simulink model "Turbulence_VonKarman"  (R2014a)
settings: Solver=ode4  StartTime=0.0  StopTime=time  FixedStep=0.02  RelTol=1e-3
PreLoadFcn:
  | load init.mat;
values from neighbouring files (symbols this model uses):
  altitude_worst = 150    [Main_turbulence_vonKarman.m]    (also in compute_variance.m)
  Vc_max = 5    [Main_turbulence_vonKarman.m]    (also in compute_variance.m)
  Vc_min = -5    [Main_turbulence_vonKarman.m]    (also in compute_variance.m)
  Vcruise = 30    [Main_turbulence_vonKarman.m]    (also in compute_variance.m)
undefined symbols (not defined in the file or in its folder): turbulenceParameters
libraries: simulink x3, aerolibconvert2 x3
settings Model: Creator=Piero  LastModifiedBy=Domenico

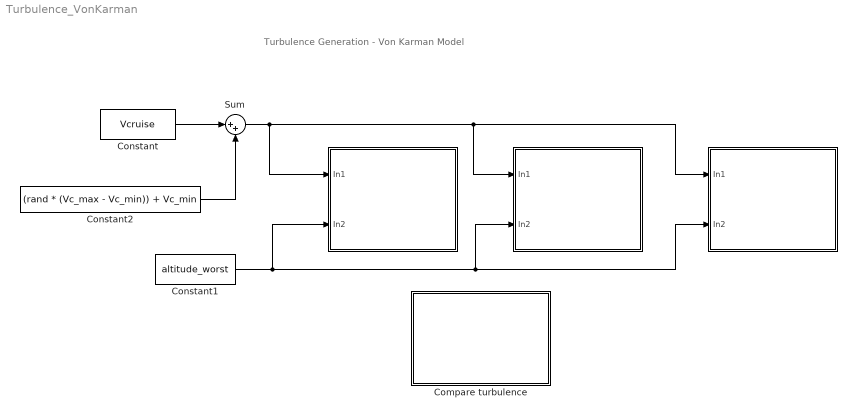
== system Turbulence_VonKarman ==
  note: Turbulence Generation - Von Karman Model
  " " : Subsystem
      mask Display:
      | color('green');
      | disp('Light Turbulence')
      | color('black');
      | port_label('input',1,'Airspeed [m/s]','texmode', 'on')
      | port_label('input',2,'Altitude [m]')
  "   " : Subsystem
      mask Display:
      | color('green');
      | disp('Moderate Turbulence')
      | color('black');
      | port_label('input',1,'Airspeed [m/s]','texmode', 'on')
      | port_label('input',2,'Altitude [m]')
  "      " : Subsystem
      mask Display:
      | color('green');
      | disp('Heavy Turbulence')
      | color('black');
      | port_label('input',1,'Airspeed [m/s]','texmode', 'on')
      | port_label('input',2,'Altitude [m]')
  " Compare turbulence" : Subsystem
      mask Display:
      | color('red');
      | disp('Plot section')
  Constant : Constant  Value=Vcruise
  Constant1 : Constant  Value=altitude_worst
  Constant2 : Constant  Value=(rand * (Vc_max - Vc_min)) + Vc_min
  Sum : Sum  Inputs=|++
  wires:
  Constant1/1 -> "      "/2(In2), "   "/2(In2), " "/2(In2)
  Sum/1 -> " "/1(In1), "   "/1(In1), "      "/1(In1)
  Constant/1 -> Sum/1
  Constant2/1 -> Sum/2

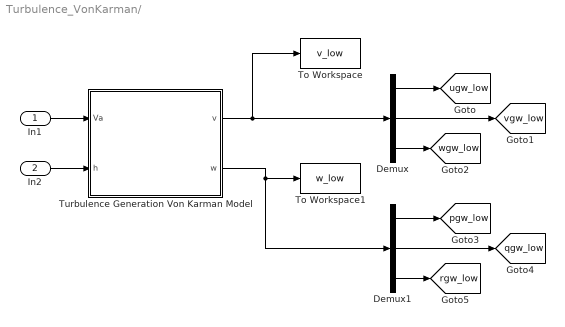
== system Turbulence_VonKarman/  ==
  In1 : Inport
  In2 : Inport  Port=2
  Demux : Demux  Outputs=3
  Demux1 : Demux  Outputs=3
  To Workspace : ToWorkspace  VariableName=v_low  SaveFormat=Structure With Time  SampleTime=-1
  To Workspace1 : ToWorkspace  VariableName=w_low  SaveFormat=Structure With Time  SampleTime=-1
  "Turbulence Generation Von Karman Model " : Subsystem  mask{ts=Light}
      mask prompts: ts "Turbulence Severity"
      mask TypeOptions ts: Light | Moderate | Heavy
      mask DialogControl DescTextVar Prompt: Generates the wind turbulences according to Dryden equations
      mask Display:
      | color('red');
      | disp('Turbulence\n Generation')
      | color('black');
      | port_label('output',1,'v_{wind}','texmode', 'on')
      | port_label('output',2,'\omega_{wind}','texmode', 'on')
      | 
      | port_label('input',1,'Airspeed')
      | port_label('input',2,'Altitude')
  tag scope: pgw_low=global, qgw_low=global, rgw_low=global, ugw_low=global, vgw_low=global, wgw_low=global
  wires:
  Demux/1 -> [ugw_low]
  Demux/2 -> [vgw_low]
  In1/1 -> "Turbulence Generation Von Karman Model "/1(Va)
  "Turbulence Generation Von Karman Model "/1(v) -> To Workspace/1, Demux/1
  "Turbulence Generation Von Karman Model "/2(w) -> To Workspace1/1, Demux1/1
  Demux1/1 -> [pgw_low]
  Demux1/2 -> [qgw_low]
  Demux1/3 -> [rgw_low]
  Demux/3 -> [wgw_low]
  In2/1 -> "Turbulence Generation Von Karman Model "/2(h)

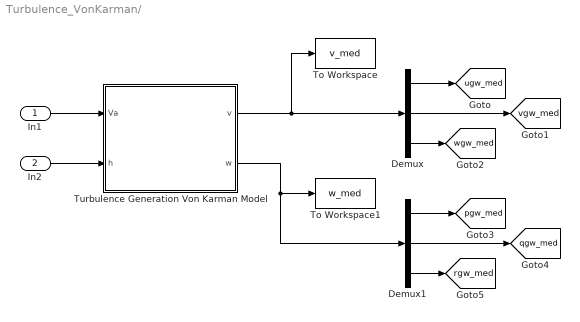
== system Turbulence_VonKarman/    ==
  In1 : Inport
  In2 : Inport  Port=2
  Demux : Demux  Outputs=3
  Demux1 : Demux  Outputs=3
  To Workspace : ToWorkspace  VariableName=v_med  SaveFormat=Structure With Time  SampleTime=-1
  To Workspace1 : ToWorkspace  VariableName=w_med  SaveFormat=Structure With Time  SampleTime=-1
  "Turbulence Generation Von Karman Model " : Subsystem  mask{ts=Moderate}
      mask prompts: ts "Turbulence Severity"
      mask TypeOptions ts: Light | Moderate | Heavy
      mask DialogControl DescTextVar Prompt: Generates the wind turbulences according to Dryden equations
      mask Display:
      | color('red');
      | disp('Turbulence\n Generation')
      | color('black');
      | port_label('output',1,'v_{wind}','texmode', 'on')
      | port_label('output',2,'\omega_{wind}','texmode', 'on')
      | 
      | port_label('input',1,'Airspeed')
      | port_label('input',2,'Altitude')
  tag scope: pgw_med=global, qgw_med=global, rgw_med=global, ugw_med=global, vgw_med=global, wgw_med=global
  wires:
  Demux/3 -> [wgw_med]
  Demux1/3 -> [rgw_med]
  Demux1/2 -> [qgw_med]
  Demux1/1 -> [pgw_med]
  "Turbulence Generation Von Karman Model "/2(w) -> To Workspace1/1, Demux1/1
  "Turbulence Generation Von Karman Model "/1(v) -> To Workspace/1, Demux/1
  Demux/2 -> [vgw_med]
  Demux/1 -> [ugw_med]
  In1/1 -> "Turbulence Generation Von Karman Model "/1(Va)
  In2/1 -> "Turbulence Generation Von Karman Model "/2(h)

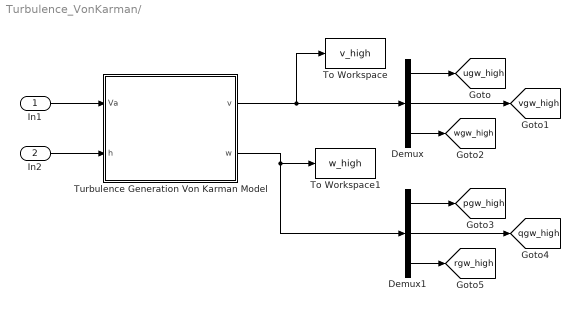
== system Turbulence_VonKarman/       ==
  In1 : Inport
  In2 : Inport  Port=2
  Demux : Demux  Outputs=3
  Demux1 : Demux  Outputs=3
  To Workspace : ToWorkspace  VariableName=v_high  SaveFormat=Structure With Time  SampleTime=-1
  To Workspace1 : ToWorkspace  VariableName=w_high  SaveFormat=Structure With Time  SampleTime=-1
  "Turbulence Generation Von Karman Model " : Subsystem  mask{ts=Heavy}
      mask prompts: ts "Turbulence Severity"
      mask TypeOptions ts: Light | Moderate | Heavy
      mask DialogControl DescTextVar Prompt: Generates the wind turbulences according to Dryden equations
      mask Display:
      | color('red');
      | disp('Turbulence\n Generation')
      | color('black');
      | port_label('output',1,'v_{wind}','texmode', 'on')
      | port_label('output',2,'\omega_{wind}','texmode', 'on')
      | 
      | port_label('input',1,'Airspeed')
      | port_label('input',2,'Altitude')
  tag scope: pgw_high=global, qgw_high=global, rgw_high=global, ugw_high=global, vgw_high=global, wgw_high=global
  wires:
  Demux/1 -> [ugw_high]
  Demux/2 -> [vgw_high]
  In2/1 -> "Turbulence Generation Von Karman Model "/2(h)
  "Turbulence Generation Von Karman Model "/1(v) -> To Workspace/1, Demux/1
  "Turbulence Generation Von Karman Model "/2(w) -> To Workspace1/1, Demux1/1
  Demux1/1 -> [pgw_high]
  Demux1/2 -> [qgw_high]
  Demux1/3 -> [rgw_high]
  Demux/3 -> [wgw_high]
  In1/1 -> "Turbulence Generation Von Karman Model "/1(Va)

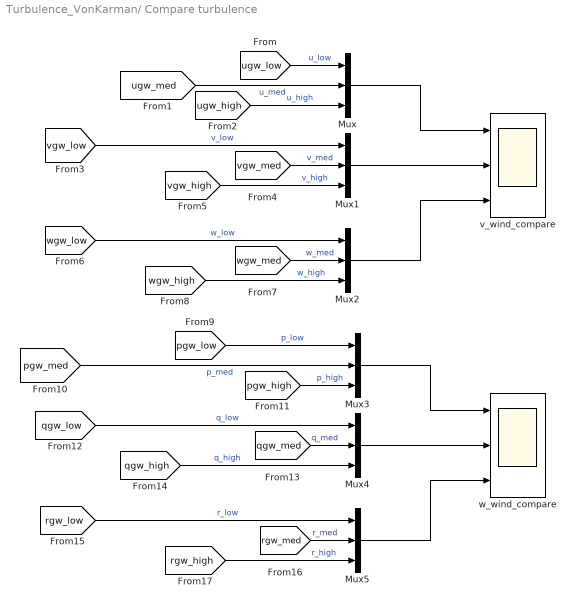
== system Turbulence_VonKarman/ Compare turbulence ==
  Mux{,1..5} (6 alike) : Mux  Inputs=3
  v_wind_compare : Scope  NumInputPorts=3
      settings: ShowLegends=on  YMin=-5~-5~-5  YMax=5~5~5  SaveName=V_wind_compare  SampleTime=0.01
  w_wind_compare : Scope  NumInputPorts=3
      settings: ShowLegends=on  YMin=-5~-5~-5  YMax=5~5~5  SaveName=w_wind_compare  SampleTime=0.01
  wires:
  [wgw_low] -> Mux2/1  "w_low"
  [ugw_med] -> Mux/2  "u_med"
  Mux/1 -> v_wind_compare/1
  [wgw_high] -> Mux2/3  "w_high"
  Mux2/1 -> v_wind_compare/3
  [vgw_med] -> Mux1/2  "v_med"
  [ugw_low] -> Mux/1  "u_low"
  [vgw_low] -> Mux1/1  "v_low"
  [vgw_high] -> Mux1/3  "v_high"
  Mux1/1 -> v_wind_compare/2
  [wgw_med] -> Mux2/2  "w_med"
  [ugw_high] -> Mux/3  "u_high"
  [qgw_med] -> Mux4/2  "q_med"
  [qgw_high] -> Mux4/3  "q_high"
  [rgw_low] -> Mux5/1  "r_low"
  [rgw_med] -> Mux5/2  "r_med"
  [rgw_high] -> Mux5/3  "r_high"
  [pgw_low] -> Mux3/1  "p_low"
  Mux3/1 -> w_wind_compare/1
  Mux4/1 -> w_wind_compare/2
  Mux5/1 -> w_wind_compare/3
  [pgw_med] -> Mux3/2  "p_med"
  [pgw_high] -> Mux3/3  "p_high"
  [qgw_low] -> Mux4/1  "q_low"

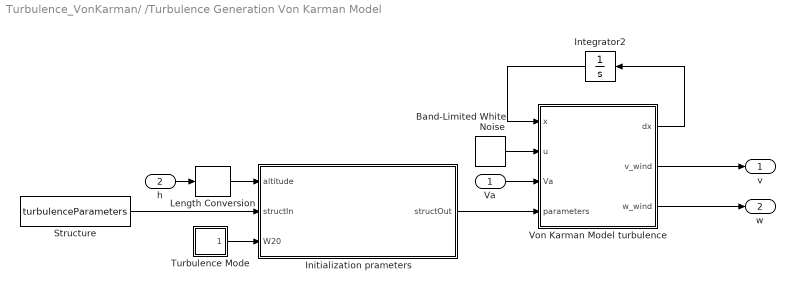
== system Turbulence_VonKarman/ /Turbulence Generation Von Karman Model  ==
  Va : Inport
  h : Inport  Port=2
  Band-Limited White Noise : simulink/Sources/Band-Limited White Noise  Cov=[0.1]  Ts=0.02  seed=[23341]
  Initialization prameters : MATLAB Function  TreatAsAtomicUnit=on
  Integrator2 : Integrator  InitialCondition=zeros(17,1)
  Length Conversion : aerolibconvert2/Length Conversion  IU=m  OU=ft
  Structure : Constant  Value=turbulenceParameters  OutDataTypeStr=Bus: myTurbParams
  Turbulence Mode : Subsystem
  Von Karman Model turbulence : MATLAB Function  TreatAsAtomicUnit=on
  v : Outport
  w : Outport  Port=2
  wires:
  h/1 -> Length Conversion/1
  Structure/1 -> Initialization prameters/2(structIn)
  Length Conversion/1 -> Initialization prameters/1(altitude)
  Va/1 -> Von Karman Model turbulence/3(Va)
  Integrator2/1 -> Von Karman Model turbulence/1(x)
  Von Karman Model turbulence/1(dx) -> Integrator2/1
  Band-Limited White Noise/1 -> Von Karman Model turbulence/2(u)
  Von Karman Model turbulence/3(w_wind) -> w/1
  Von Karman Model turbulence/2(v_wind) -> v/1
  Initialization prameters/1(structOut) -> Von Karman Model turbulence/4(parameters)
  Turbulence Mode/1(W20) -> Initialization prameters/3(W20)

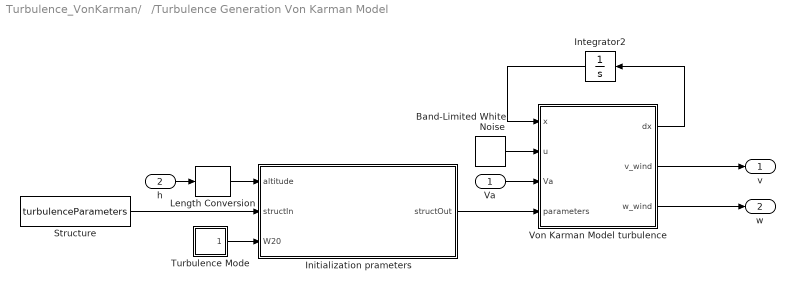
== system Turbulence_VonKarman/   /Turbulence Generation Von Karman Model  ==
  Va : Inport
  h : Inport  Port=2
  Band-Limited White Noise : simulink/Sources/Band-Limited White Noise  Cov=[0.1]  Ts=0.02  seed=[23341]
  Initialization prameters : MATLAB Function  TreatAsAtomicUnit=on
  Integrator2 : Integrator  InitialCondition=zeros(17,1)
  Length Conversion : aerolibconvert2/Length Conversion  IU=m  OU=ft
  Structure : Constant  Value=turbulenceParameters  OutDataTypeStr=Bus: myTurbParams
  Turbulence Mode : Subsystem
  Von Karman Model turbulence : MATLAB Function  TreatAsAtomicUnit=on
  v : Outport
  w : Outport  Port=2
  wires:
  Turbulence Mode/1(W20) -> Initialization prameters/3(W20)
  Initialization prameters/1(structOut) -> Von Karman Model turbulence/4(parameters)
  Von Karman Model turbulence/2(v_wind) -> v/1
  Von Karman Model turbulence/3(w_wind) -> w/1
  Band-Limited White Noise/1 -> Von Karman Model turbulence/2(u)
  Von Karman Model turbulence/1(dx) -> Integrator2/1
  Integrator2/1 -> Von Karman Model turbulence/1(x)
  Va/1 -> Von Karman Model turbulence/3(Va)
  Length Conversion/1 -> Initialization prameters/1(altitude)
  Structure/1 -> Initialization prameters/2(structIn)
  h/1 -> Length Conversion/1

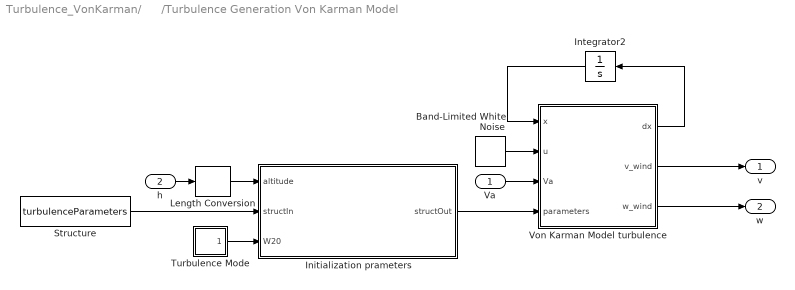
== system Turbulence_VonKarman/      /Turbulence Generation Von Karman Model  ==
  Va : Inport
  h : Inport  Port=2
  Band-Limited White Noise : simulink/Sources/Band-Limited White Noise  Cov=[0.1]  Ts=0.02  seed=[23341]
  Initialization prameters : MATLAB Function  TreatAsAtomicUnit=on
  Integrator2 : Integrator  InitialCondition=zeros(17,1)
  Length Conversion : aerolibconvert2/Length Conversion  IU=m  OU=ft
  Structure : Constant  Value=turbulenceParameters  OutDataTypeStr=Bus: myTurbParams
  Turbulence Mode : Subsystem
  Von Karman Model turbulence : MATLAB Function  TreatAsAtomicUnit=on
  v : Outport
  w : Outport  Port=2
  wires:
  h/1 -> Length Conversion/1
  Structure/1 -> Initialization prameters/2(structIn)
  Length Conversion/1 -> Initialization prameters/1(altitude)
  Va/1 -> Von Karman Model turbulence/3(Va)
  Integrator2/1 -> Von Karman Model turbulence/1(x)
  Von Karman Model turbulence/1(dx) -> Integrator2/1
  Band-Limited White Noise/1 -> Von Karman Model turbulence/2(u)
  Von Karman Model turbulence/3(w_wind) -> w/1
  Von Karman Model turbulence/2(v_wind) -> v/1
  Initialization prameters/1(structOut) -> Von Karman Model turbulence/4(parameters)
  Turbulence Mode/1(W20) -> Initialization prameters/3(W20)

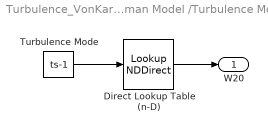
== system Turbulence_VonKarman/ /Turbulence Generation Von Karman Model /Turbulence Mode ==
  Direct Lookup Table (n-D) : LookupNDDirect  NumberOfTableDimensions=1  Table=[15 30 45]
  Turbulence Mode : Constant  Value=ts-1
  W20 : Outport
  wires:
  Direct Lookup Table (n-D)/1 -> W20/1
  Turbulence Mode/1 -> Direct Lookup Table (n-D)/1

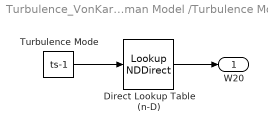
== system Turbulence_VonKarman/   /Turbulence Generation Von Karman Model /Turbulence Mode ==
  Direct Lookup Table (n-D) : LookupNDDirect  NumberOfTableDimensions=1  Table=[15 30 45]
  Turbulence Mode : Constant  Value=ts-1
  W20 : Outport
  wires:
  Turbulence Mode/1 -> Direct Lookup Table (n-D)/1
  Direct Lookup Table (n-D)/1 -> W20/1

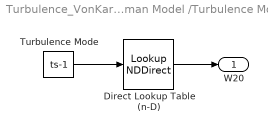
== system Turbulence_VonKarman/      /Turbulence Generation Von Karman Model /Turbulence Mode ==
  Direct Lookup Table (n-D) : LookupNDDirect  NumberOfTableDimensions=1  Table=[15 30 45]
  Turbulence Mode : Constant  Value=ts-1
  W20 : Outport
  wires:
  Direct Lookup Table (n-D)/1 -> W20/1
  Turbulence Mode/1 -> Direct Lookup Table (n-D)/1

== matlab function Turbulence_VonKarman/      /Turbulence Generation Von Karman Model /Initialization prameters ==
  data: altitude input; structOut output Bus: myTurbParams; structIn input; W20 input
function structOut = initTurbulenceParameters( altitude , structIn , W20 )
%initTurbulenceParameters returns scale lengths and turbulence intensities
%parameters depending of altitude of aircraft and also of turbolence severity
%in case of low altitude (h<1000ft)

%   Form: initTurbulenceParameters( altitude, modeTurb )
%   Inputs :    altitude             -> altitude of aircraft [m]
%               modeTurbolence       -> turbolence severity
%               turbolenceParameters -> structure of parameters 
%   Outputs :   turbolenceParameters -> Lu,Lv,Lw,sigma_u,sigma_v,sigma_w

% LOW ALTITUDE (h<1000ft)
if(altitude>0 && altitude<=1000)
Lw=altitude;
Lu=altitude/((0.177+0.000823*altitude)^(1.2));
Lv=Lu;

sigma_w=0.1*W20; %suppose 10% of probability of exceedence
sigma_u=sigma_w/((0.177+0.000823*altitude)^(0.4));
sigma_v=sigma_u;

elseif(altitude>=2000) % MEDIUM/HIGH ALTITUDE (h>2000ft)
Lw=2500;
Lu=Lw;
Lv=Lw;
sigma_w=0.2*W20; %suppose 20% of probability of exceedence
sigma_u=sigma_w;
sigma_v=sigma_w;

elseif(altitude>1000 && altitude<2000)% LOW/MEDIUM ALTITUDE (1000ft<h<2000ft)
LwLOW=altitude;
LuLOW=altitude/((0.177+0.000823*altitude)^(1.2));
LvLOW=LuLOW;
sigma_wLOW=0.1*W20;
sigma_uLOW=sigma_wLOW/((0.177+0.000823*altitude)^(0.4));
sigma_vLOW=sigma_uLOW;
LwHIGH=2500;
LuHIGH=LwHIGH;
LvHIGH=LwHIGH;

sigma_wHIGH=0.2*W20; 
sigma_uHIGH=sigma_wHIGH;
sigma_vHIGH=sigma_wHIGH;
Lw=mean([LwLOW,LwHIGH ]);
Lu=mean([LuLOW,LuHIGH ]);
Lv=mean([LvLOW,LvHIGH ]);

sigma_w=mean([sigma_wLOW,sigma_wHIGH ]);
sigma_u=mean([sigma_uLOW,sigma_uHIGH ]);
sigma_v=mean([sigma_vLOW,sigma_vHIGH ]);

else
Lw=0;
Lu=0;
Lv=0;
sigma_w=0;
sigma_u=0;
sigma_v=0;
end

structIn.Lu       = Lu;
structIn.Lv       = Lv;
structIn.Lw       = Lw;
structIn.sigma_u  = sigma_u;
structIn.sigma_v  = sigma_v;
structIn.sigma_w  = sigma_w;

structOut = structIn;
end

== matlab function Turbulence_VonKarman/ /Turbulence Generation Von Karman Model /Initialization prameters ==
  data: altitude input; structOut output Bus: myTurbParams; structIn input; W20 input
function structOut  = initTurbulenceParameters( altitude , structIn , W20 )
%initTurbulenceParameters returns scale lengths and turbulence intensities
%parameters depending of altitude of aircraft and also of turbolence severity
%in case of low altitude (h<1000ft)

%   Form: initTurbulenceParameters( altitude, modeTurb )
%   Inputs :    altitude             -> altitude of aircraft [m]
%               modeTurbolence       -> turbolence severity
%               turbolenceParameters -> structure of parameters 
%   Outputs :   turbolenceParameters -> Lu,Lv,Lw,sigma_u,sigma_v,sigma_w


% LOW ALTITUDE (h<1000ft)
if(altitude>0 && altitude<=1000)
Lw=altitude;
Lu=altitude/((0.177+0.000823*altitude)^(1.2));
Lv=Lu;

sigma_w=0.1*W20; %suppose 10% of probability of exceedence
sigma_u=sigma_w/((0.177+0.000823*altitude)^(0.4));
sigma_v=sigma_u;

elseif(altitude>=2000) % MEDIUM/HIGH ALTITUDE (h>2000ft)
Lw=2500;
Lu=Lw;
Lv=Lw;
sigma_w=0.2*W20; %suppose 20% of probability of exceedence
sigma_u=sigma_w;
sigma_v=sigma_w;

elseif(altitude>1000 && altitude<2000)% LOW/MEDIUM ALTITUDE (1000ft<h<2000ft)
LwLOW=altitude;
LuLOW=altitude/((0.177+0.000823*altitude)^(1.2));
LvLOW=LuLOW;
sigma_wLOW=0.1*W20;
sigma_uLOW=sigma_wLOW/((0.177+0.000823*altitude)^(0.4));
sigma_vLOW=sigma_uLOW;
LwHIGH=2500;
LuHIGH=LwHIGH;
LvHIGH=LwHIGH;

sigma_wHIGH=0.2*W20; 
sigma_uHIGH=sigma_wHIGH;
sigma_vHIGH=sigma_wHIGH;
Lw=mean([LwLOW,LwHIGH ]);
Lu=mean([LuLOW,LuHIGH ]);
Lv=mean([LvLOW,LvHIGH ]);

sigma_w=mean([sigma_wLOW,sigma_wHIGH ]);
sigma_u=mean([sigma_uLOW,sigma_uHIGH ]);
sigma_v=mean([sigma_vLOW,sigma_vHIGH ]);

else
Lw=0;
Lu=0;
Lv=0;
sigma_w=0;
sigma_u=0;
sigma_v=0;
end

structIn.Lu       = Lu;
structIn.Lv       = Lv;
structIn.Lw       = Lw;
structIn.sigma_u  = sigma_u;
structIn.sigma_v  = sigma_v;
structIn.sigma_w  = sigma_w;

structOut = structIn;
end

== matlab function Turbulence_VonKarman/ /Turbulence Generation Von Karman Model /Von Karman Model turbulence ==
  data: x input; u input; dx output; v_wind output; w_wind output; Va input; parameters input Bus: myTurbParams
function [dx,v_wind,w_wind]  = fcn(x,u,Va,parameters)
%This function returns V_wind and w_wind vectors by linear and angular
%velocity of wind - Von-Karman Model

%   Form: fcn(x,u,parameters,V)
%   Inputs :    x              -> state
%               u              -> white noise
%               parameters     -> vector parameters
%               V              -> velocity aircraft
%   Outputs :   V_wind         -> linear speed wind [u,v,w]
%               w_wind         -> angular rate wind [p,q,r]
%               dx             -> differential state

%% State component
ux   = x(1); % longitudinal u-component (TRANSLATIONAL COMPONENT)
uxd  = x(2); % derived u-component
vx   = x(3); % lateral v-component (TRANSLATIONAL COMPONENT)
vxd  = x(4); % derived v-component
vx2d = x(5); % second derived of v-component
wx   = x(6); % vertical w-component(TRANSLATIONAL COMPONENT)
wxd  = x(7); % derived w-component
wx2d = x(8); % second derived of w-component
px   = x(9); % Longitudinal p-component (ROTATIONAL COMPONENT)
rx   = x(10); % Lateral r-component (ROTATIONAL COMPONENT)
rxd  = x(11); % derived of r-component
rx2d = x(12); % second derived of r-component
rx3d = x(13); % third derived of r-component
qx   = x(14);% vertical q-component (ROTATIONAL COMPONENT)
qxd  = x(15);% derived of p-component
qx2d = x(16);% second derived of p-component
qx3d = x(17);% third derived of p-component
%% Input 
eta = u; % white noise

%% Parameters
% %turbolence intensities
sigma_u = parameters.sigma_u;
sigma_v = parameters.sigma_v;
sigma_w = parameters.sigma_w;
% %scale lengths
Lu      = parameters.Lu;
Lv      = parameters.Lv;
Lw      = parameters.Lw;
b       = 4.5; %wing span

%% Util terms
Va=abs(Va);

a1Term = sigma_u*sqrt(2/pi*Lu/Va);
b1Term = 0.25*Lu/Va;
c1Term = 1.357*Lu/Va;
d1Term = 0.1987 *(Lu/Va)^2;
a2Term = sigma_v*sqrt(1/pi*Lv/Va);
b2Term = 2.7478*Lv/Va;
c2Term = 0.3398*(Lv/Va)^2;
d2Term = 2.9958*Lv/Va;
e2Term = 1.9754*(Lv/Va)^2;
f2Term = 0.1539*(Lv/Va)^3;
a3Term = sigma_w*sqrt(1/pi*Lw/Va);
b3Term = 2.7478*Lw/Va;
c3Term = 0.3398*(Lw/Va)^2;
d3Term = 2.9958*Lw/Va;
e3Term = 1.9754*(Lw/Va)^2;
f3Term = 0.1539*(Lw/Va)^3;
a4Term = (sigma_w*sqrt(0.8/Va)*(pi/(4*b)^(1/6)))/(Lw^(1/3));
b4Term = (4*b)/(pi*Va);
a5Term = (3*b)/(pi*Va);

dx=[uxd;
   -(ux/d1Term) - ((c1Term*uxd)/d1Term)+ eta;
   vxd;
   vx2d;
   -(vx/f2Term) - ((d2Term*vxd)/f2Term) - ((e2Term*vx2d)/f2Term) + eta;
   wxd;
   wx2d;
   -(wx/f3Term) - ((d3Term*wxd)/f3Term) - ((e3Term*wx2d)/f3Term) + eta;
   -px/b4Term+eta;
   rxd;
   rx2d;
   rx3d;
   eta-(rx/(f2Term*a5Term))-((a2Term+a5Term)*rxd)/(f2Term*a5Term)-((e2Term+d2Term*a5Term)*rx2d)/(f2Term*a5Term)-((f2Term+e2Term*a5Term)*rx3d)/(f2Term*a5Term);
   qxd;
   qx2d;
   qx3d;
   eta-(qx/(f3Term*b4Term))-((a3Term+b4Term)*qxd)/(f3Term*b4Term)-((e3Term+d3Term*b4Term)*qx2d)/(f3Term*b4Term)-((f3Term+e3Term*b4Term)*qx3d)/(f3Term*b4Term)];
 

%% Translational component of wind 
ugw = (a1Term/d1Term)*ux+((a1Term*b1Term)/d1Term)*uxd;                                   % Longitudinal
vgw = (a2Term/f2Term)*vx+((a2Term*b2Term)/f2Term)*vxd+((a2Term*c2Term)/f2Term)*vx2d;     % Lateral
wgw = (a3Term/f3Term)*wx+((a3Term*b3Term)/f3Term)*wxd+((a3Term*c3Term)/f3Term)*wx2d;     % Vertical

%% Rotational component of wind 
pgw = (a4Term/b4Term)*px;                                                                                                 % Longitudinal
rgw = (a2Term/(f2Term*a5Term*Va))*rxd+((a2Term*b2Term)/(f2Term*a5Term*Va))*rx2d + ((a2Term*c2Term)/(f2Term*a5Term*Va))*rx3d;  % Lateral
qgw = (a3Term/(f3Term*b4Term*Va))*qxd+((a3Term*b3Term)/(f3Term*b4Term*Va))*qx2d + ((a3Term*c3Term)/(f3Term*b4Term*Va))*qx3d;   % Vertical

v_wind=[ugw;vgw;wgw];
w_wind=[pgw;qgw;rgw];

== matlab function Turbulence_VonKarman/      /Turbulence Generation Von Karman Model /Von Karman Model turbulence ==
  data: x input; u input; dx output; v_wind output; w_wind output; Va input; parameters input Bus: myTurbParams
function [dx,v_wind,w_wind]  = fcn(x,u,Va,parameters)
%This function returns V_wind and w_wind vectors by linear and angular
%velocity of wind - Von-Karman Model

%   Form: fcn(x,u,parameters,V)
%   Inputs :    x              -> state
%               u              -> white noise
%               parameters     -> vector parameters
%               V              -> velocity aircraft
%   Outputs :   V_wind         -> linear speed wind [u,v,w]
%               w_wind         -> angular rate wind [p,q,r]
%               dx             -> differential state

%% State component
ux   = x(1); % longitudinal u-component (TRANSLATIONAL COMPONENT)
uxd  = x(2); % derived u-component
vx   = x(3); % lateral v-component (TRANSLATIONAL COMPONENT)
vxd  = x(4); % derived v-component
vx2d = x(5); % second derived of v-component
wx   = x(6); % vertical w-component(TRANSLATIONAL COMPONENT)
wxd  = x(7); % derived w-component
wx2d = x(8); % second derived of w-component
px   = x(9); % Longitudinal p-component (ROTATIONAL COMPONENT)
rx   = x(10); % Lateral r-component (ROTATIONAL COMPONENT)
rxd  = x(11); % derived of r-component
rx2d = x(12); % second derived of r-component
rx3d = x(13); % third derived of r-component
qx   = x(14);% vertical q-component (ROTATIONAL COMPONENT)
qxd  = x(15);% derived of p-component
qx2d = x(16);% second derived of p-component
qx3d = x(17);% third derived of p-component
%% Input 
eta = u; % white noise

%% Parameters
% %turbolence intensities
sigma_u = parameters.sigma_u;
sigma_v = parameters.sigma_v;
sigma_w = parameters.sigma_w;
% %scale lengths
Lu      = parameters.Lu;
Lv      = parameters.Lv;
Lw      = parameters.Lw;
b       = 4.5; %wing span

%% Util terms
Va=abs(Va);

a1Term = sigma_u*sqrt(2/pi*Lu/Va);
b1Term = 0.25*Lu/Va;
c1Term = 1.357*Lu/Va;
d1Term = 0.1987 *(Lu/Va)^2;
a2Term = sigma_v*sqrt(1/pi*Lv/Va);
b2Term = 2.7478*Lv/Va;
c2Term = 0.3398*(Lv/Va)^2;
d2Term = 2.9958*Lv/Va;
e2Term = 1.9754*(Lv/Va)^2;
f2Term = 0.1539*(Lv/Va)^3;
a3Term = sigma_w*sqrt(1/pi*Lw/Va);
b3Term = 2.7478*Lw/Va;
c3Term = 0.3398*(Lw/Va)^2;
d3Term = 2.9958*Lw/Va;
e3Term = 1.9754*(Lw/Va)^2;
f3Term = 0.1539*(Lw/Va)^3;
a4Term = (sigma_w*sqrt(0.8/Va)*(pi/(4*b)^(1/6)))/(Lw^(1/3));
b4Term = (4*b)/(pi*Va);
a5Term = (3*b)/(pi*Va);

dx=[uxd;
   -(ux/d1Term) - ((c1Term*uxd)/d1Term)+ eta;
   vxd;
   vx2d;
   -(vx/f2Term) - ((d2Term*vxd)/f2Term) - ((e2Term*vx2d)/f2Term) + eta;
   wxd;
   wx2d;
   -(wx/f3Term) - ((d3Term*wxd)/f3Term) - ((e3Term*wx2d)/f3Term) + eta;
   -px/b4Term+eta;
   rxd;
   rx2d;
   rx3d;
   eta-(rx/(f2Term*a5Term))-((a2Term+a5Term)*rxd)/(f2Term*a5Term)-((e2Term+d2Term*a5Term)*rx2d)/(f2Term*a5Term)-((f2Term+e2Term*a5Term)*rx3d)/(f2Term*a5Term);
   qxd;
   qx2d;
   qx3d;
   eta-(qx/(f3Term*b4Term))-((a3Term+b4Term)*qxd)/(f3Term*b4Term)-((e3Term+d3Term*b4Term)*qx2d)/(f3Term*b4Term)-((f3Term+e3Term*b4Term)*qx3d)/(f3Term*b4Term)];
 

%% Translational component of wind 
ugw = (a1Term/d1Term)*ux+((a1Term*b1Term)/d1Term)*uxd;                                   % Longitudinal
vgw = (a2Term/f2Term)*vx+((a2Term*b2Term)/f2Term)*vxd+((a2Term*c2Term)/f2Term)*vx2d;     % Lateral
wgw = (a3Term/f3Term)*wx+((a3Term*b3Term)/f3Term)*wxd+((a3Term*c3Term)/f3Term)*wx2d;     % Vertical

%% Rotational component of wind 
pgw = (a4Term/b4Term)*px;                                                                                                 % Longitudinal
rgw = (a2Term/(f2Term*a5Term*Va))*rxd+((a2Term*b2Term)/(f2Term*a5Term*Va))*rx2d + ((a2Term*c2Term)/(f2Term*a5Term*Va))*rx3d;  % Lateral
qgw = (a3Term/(f3Term*b4Term*Va))*qxd+((a3Term*b3Term)/(f3Term*b4Term*Va))*qx2d + ((a3Term*c3Term)/(f3Term*b4Term*Va))*qx3d;   % Vertical

v_wind=[ugw;vgw;wgw];
w_wind=[pgw;qgw;rgw];

== matlab function Turbulence_VonKarman/   /Turbulence Generation Von Karman Model /Initialization prameters ==
  data: altitude input; structOut output Bus: myTurbParams; structIn input; W20 input
function structOut = initTurbulenceParameters( altitude , structIn , W20 )
%initTurbulenceParameters returns scale lengths and turbulence intensities
%parameters depending of altitude of aircraft and also of turbolence severity
%in case of low altitude (h<1000ft)

%   Form: initTurbulenceParameters( altitude, modeTurb )
%   Inputs :    altitude             -> altitude of aircraft [m]
%               modeTurbolence       -> turbolence severity
%               turbolenceParameters -> structure of parameters 
%   Outputs :   turbolenceParameters -> Lu,Lv,Lw,sigma_u,sigma_v,sigma_w

% LOW ALTITUDE (h<1000ft)
if(altitude>0 && altitude<=1000)
Lw=altitude;
Lu=altitude/((0.177+0.000823*altitude)^(1.2));
Lv=Lu;

sigma_w=0.1*W20; %suppose 10% of probability of exceedence
sigma_u=sigma_w/((0.177+0.000823*altitude)^(0.4));
sigma_v=sigma_u;

elseif(altitude>=2000) % MEDIUM/HIGH ALTITUDE (h>2000ft)
Lw=2500;
Lu=Lw;
Lv=Lw;
sigma_w=0.2*W20; %suppose 20% of probability of exceedence
sigma_u=sigma_w;
sigma_v=sigma_w;

elseif(altitude>1000 && altitude<2000)% LOW/MEDIUM ALTITUDE (1000ft<h<2000ft)
LwLOW=altitude;
LuLOW=altitude/((0.177+0.000823*altitude)^(1.2));
LvLOW=LuLOW;
sigma_wLOW=0.1*W20;
sigma_uLOW=sigma_wLOW/((0.177+0.000823*altitude)^(0.4));
sigma_vLOW=sigma_uLOW;
LwHIGH=2500;
LuHIGH=LwHIGH;
LvHIGH=LwHIGH;

sigma_wHIGH=0.2*W20; 
sigma_uHIGH=sigma_wHIGH;
sigma_vHIGH=sigma_wHIGH;
Lw=mean([LwLOW,LwHIGH ]);
Lu=mean([LuLOW,LuHIGH ]);
Lv=mean([LvLOW,LvHIGH ]);


sigma_w=mean([sigma_wLOW,sigma_wHIGH ]);
sigma_u=mean([sigma_uLOW,sigma_uHIGH ]);
sigma_v=mean([sigma_vLOW,sigma_vHIGH ]);

else
Lw=0;
Lu=0;
Lv=0;
sigma_w=0;
sigma_u=0;
sigma_v=0;
end

structIn.Lu       = Lu;
structIn.Lv       = Lv;
structIn.Lw       = Lw;
structIn.sigma_u  = sigma_u;
structIn.sigma_v  = sigma_v;
structIn.sigma_w  = sigma_w;

structOut = structIn;
end

== matlab function Turbulence_VonKarman/   /Turbulence Generation Von Karman Model /Von Karman Model turbulence ==
  data: x input; u input; dx output; v_wind output; w_wind output; Va input; parameters input Bus: myTurbParams
function [dx,v_wind,w_wind]  = fcn(x,u,Va,parameters)
%This function returns V_wind and w_wind vectors by linear and angular
%velocity of wind - Von-Karman Model

%   Form: fcn(x,u,parameters,V)
%   Inputs :    x              -> state
%               u              -> white noise
%               parameters     -> vector parameters
%               V              -> velocity aircraft
%   Outputs :   V_wind         -> linear speed wind [u,v,w]
%               w_wind         -> angular rate wind [p,q,r]
%               dx             -> differential state

%% State component
ux   = x(1); % longitudinal u-component (TRANSLATIONAL COMPONENT)
uxd  = x(2); % derived u-component
vx   = x(3); % lateral v-component (TRANSLATIONAL COMPONENT)
vxd  = x(4); % derived v-component
vx2d = x(5); % second derived of v-component
wx   = x(6); % vertical w-component(TRANSLATIONAL COMPONENT)
wxd  = x(7); % derived w-component
wx2d = x(8); % second derived of w-component
px   = x(9); % Longitudinal p-component (ROTATIONAL COMPONENT)
rx   = x(10); % Lateral r-component (ROTATIONAL COMPONENT)
rxd  = x(11); % derived of r-component
rx2d = x(12); % second derived of r-component
rx3d = x(13); % third derived of r-component
qx   = x(14);% vertical q-component (ROTATIONAL COMPONENT)
qxd  = x(15);% derived of p-component
qx2d = x(16);% second derived of p-component
qx3d = x(17);% third derived of p-component
%% Input 
eta = u; % white noise

%% Parameters
% %turbolence intensities
sigma_u = parameters.sigma_u;
sigma_v = parameters.sigma_v;
sigma_w = parameters.sigma_w;
% %scale lengths
Lu      = parameters.Lu;
Lv      = parameters.Lv;
Lw      = parameters.Lw;
b       = 4.5; %wing span

%% Util terms
Va=abs(Va);

a1Term = sigma_u*sqrt(2/pi*Lu/Va);
b1Term = 0.25*Lu/Va;
c1Term = 1.357*Lu/Va;
d1Term = 0.1987 *(Lu/Va)^2;
a2Term = sigma_v*sqrt(1/pi*Lv/Va);
b2Term = 2.7478*Lv/Va;
c2Term = 0.3398*(Lv/Va)^2;
d2Term = 2.9958*Lv/Va;
e2Term = 1.9754*(Lv/Va)^2;
f2Term = 0.1539*(Lv/Va)^3;
a3Term = sigma_w*sqrt(1/pi*Lw/Va);
b3Term = 2.7478*Lw/Va;
c3Term = 0.3398*(Lw/Va)^2;
d3Term = 2.9958*Lw/Va;
e3Term = 1.9754*(Lw/Va)^2;
f3Term = 0.1539*(Lw/Va)^3;
a4Term = (sigma_w*sqrt(0.8/Va)*(pi/(4*b)^(1/6)))/(Lw^(1/3));
b4Term = (4*b)/(pi*Va);
a5Term = (3*b)/(pi*Va);

dx=[uxd;
   -(ux/d1Term) - ((c1Term*uxd)/d1Term)+ eta;
   vxd;
   vx2d;
   -(vx/f2Term) - ((d2Term*vxd)/f2Term) - ((e2Term*vx2d)/f2Term) + eta;
   wxd;
   wx2d;
   -(wx/f3Term) - ((d3Term*wxd)/f3Term) - ((e3Term*wx2d)/f3Term) + eta;
   -px/b4Term+eta;
   rxd;
   rx2d;
   rx3d;
   eta-(rx/(f2Term*a5Term))-((a2Term+a5Term)*rxd)/(f2Term*a5Term)-((e2Term+d2Term*a5Term)*rx2d)/(f2Term*a5Term)-((f2Term+e2Term*a5Term)*rx3d)/(f2Term*a5Term);
   qxd;
   qx2d;
   qx3d;
   eta-(qx/(f3Term*b4Term))-((a3Term+b4Term)*qxd)/(f3Term*b4Term)-((e3Term+d3Term*b4Term)*qx2d)/(f3Term*b4Term)-((f3Term+e3Term*b4Term)*qx3d)/(f3Term*b4Term)];
 

%% Translational component of wind 
ugw = (a1Term/d1Term)*ux+((a1Term*b1Term)/d1Term)*uxd;                                   % Longitudinal
vgw = (a2Term/f2Term)*vx+((a2Term*b2Term)/f2Term)*vxd+((a2Term*c2Term)/f2Term)*vx2d;     % Lateral
wgw = (a3Term/f3Term)*wx+((a3Term*b3Term)/f3Term)*wxd+((a3Term*c3Term)/f3Term)*wx2d;     % Vertical

%% Rotational component of wind 
pgw = (a4Term/b4Term)*px;                                                                                                 % Longitudinal
rgw = (a2Term/(f2Term*a5Term*Va))*rxd+((a2Term*b2Term)/(f2Term*a5Term*Va))*rx2d + ((a2Term*c2Term)/(f2Term*a5Term*Va))*rx3d;  % Lateral
qgw = (a3Term/(f3Term*b4Term*Va))*qxd+((a3Term*b3Term)/(f3Term*b4Term*Va))*qx2d + ((a3Term*c3Term)/(f3Term*b4Term*Va))*qx3d;   % Vertical

v_wind=[ugw;vgw;wgw];
w_wind=[pgw;qgw;rgw];
